simulink model "dynamics"  (R2025b)
settings: Solver=ode3  StartTime=0.0  StopTime=inf  FixedStep=0.015  RelTol=1e-3
settings Model: Creator=brusie  LastModifiedBy=brusie

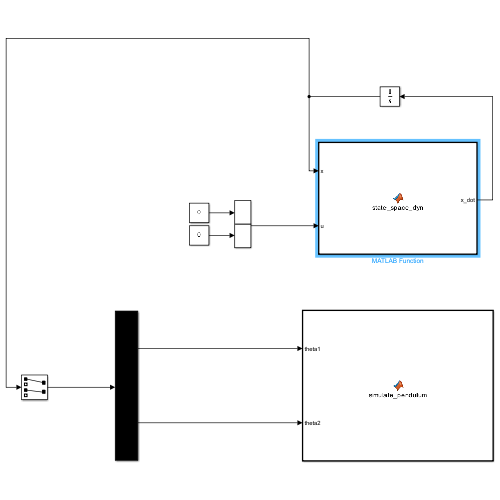
[thumbnail: Simulink's stored preview of the top-level diagram]
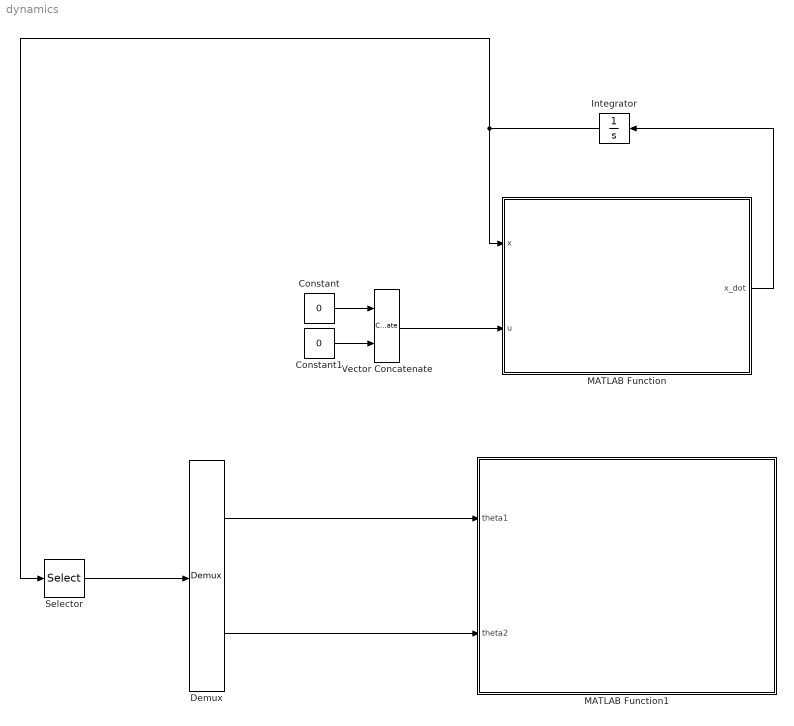
== system dynamics ==
  Constant : Constant  Value=0
  Constant1 : Constant  Value=0
  Demux : Demux  Outputs=2
  Integrator : Integrator  InitialCondition=[0,0,0.1,0]'
  MATLAB Function : MATLAB Function  TreatAsAtomicUnit=on
  MATLAB Function1 : MATLAB Function  TreatAsAtomicUnit=on
  Selector : Selector  InputPortWidth=4  IndexOptions=Index vector (dialog)  Indices=[1 3]  OutputSizes=1
  Vector Concatenate : Concatenate
  wires:
  MATLAB Function/1(x_dot) -> Integrator/1
  Integrator/1 -> MATLAB Function/1(x), Selector/1
  Selector/1 -> Demux/1
  Demux/1 -> MATLAB Function1/1(theta1)
  Demux/2 -> MATLAB Function1/2(theta2)
  Vector Concatenate/1 -> MATLAB Function/2(u)
  Constant/1 -> Vector Concatenate/1
  Constant1/1 -> Vector Concatenate/2

== matlab function dynamics/MATLAB Function ==
  data: x input; u input; x_dot output
function x_dot = state_space_dyn(x, u)
    q = [x(1); x(3)];
    qd = [x(2); x(4)];
    v = u;

    %Ra = 2.6;
    %b1 = 0.015;
    %b2 = 0.002;
    %kt = 0.00768;
    %kv = 0.00768;
    
    %l1 = 0.2;
    %l2 = 0.3;
    %J1 = 0.0012;
    %m2 = 0.127;
    %kr = 70;
    %lc2 = 0.15;
    %v2 = 0;
    
    % parameters t is \theta
    %t1p = J1 + m2*(l1+l2);
    %t2p = 1/3*m2*l2^2;
    %t3p = 1/2*m2*(l1)*l2;
    %t4p = m2*lc2;
    
    % parameter theta 1~6
    t1 = 0.3129;   
    t2 = 0.0184;
    t3 = 0.0184;
    t4 = 0.0921;
    t5 = 0.6101;
    t6 = 0.0097;

    

    q1 = q(1);
    q2 = q(2);
    dq1 = qd(1);
    dq2 = qd(2);


    M = [t1+t2*sin(q2)^2 t3*cos(q2);
        t3*cos(q2) t2];


    C = [2*t2*sin(q2)*cos(q2)*dq2 -t3*sin(q2)*dq2;
         -t2*sin(q2)*cos(q2)*dq1    0];
    
    f = [t5*dq1; t6*dq2];
    
    g = [0; -t4*sin(q2)];

    qdd = M\(v-C*qd-f-g);

    x_dot = [qd(1); qdd(1); qd(2); qdd(2)];

== matlab function dynamics/MATLAB Function1 ==
  data: theta1 input; theta2 input
function simulate_pendulum(theta1, theta2)

    d = 8;
    % link 2 (in its own frame) - forearm
    p1 = [0,0,0];
    p2 = [0,12,0];
    link2_frame2 = [p1' p2'; ones(1,2)];
    
    % link 1 (in its own frame) - bicep
    pts = [0, 0, 0, 0, 0;
           0, 0, 6, 6, 8;
           0, -1, -1, 0, 0];
    link1_frame1 = [pts; ones(1,5)];
    full_model_frame0 = [TRANS0_1(link1_frame1, theta1), TRANS0_1(TRANS1_2(link2_frame2, theta2, d), theta1)];


    % PLOT ROBOT
    pointsorg = full_model_frame0;
    s = 1;
    g = 7; % total num of points
    plot3(pointsorg(1,s:g), pointsorg(2,s:g), pointsorg(3,s:g), 'LineWidth',3);
    axis equal;
    xlim([-20 20]);
    ylim([-20 20]);
    zlim([-20 20]);

    grid on;


end

function points_frame1 = TRANS1_2(link2_frame2, theta2,d) % this is task 5

    t2_1 = [cos(theta2) -sin(theta2)       0       0;
              0                   0        -1       d;
            sin(theta2)  cos(theta2)        0       0;
                0                0            0       1];

    points_frame1 = t2_1*link2_frame2;



end

function points_frame0 = TRANS0_1(link1_frame1, theta1) % this is task 3

    t1_0 = [cos(theta1) -sin(theta1)       0       0;
     sin(theta1) cos(theta1)        0        0;
     0           0            1            0;
     0             0        0              1];

    points_frame0 = t1_0*link1_frame1;


end
